simulink model "model_mavic_attitude_pid"  (R2020b)
settings: Solver=VariableStepAuto  StartTime=0.0  StopTime=10.0  RelTol=1e-3
libraries: pid_lib x1
settings Model: Creator=boringtao  LastModifiedBy=boringtao

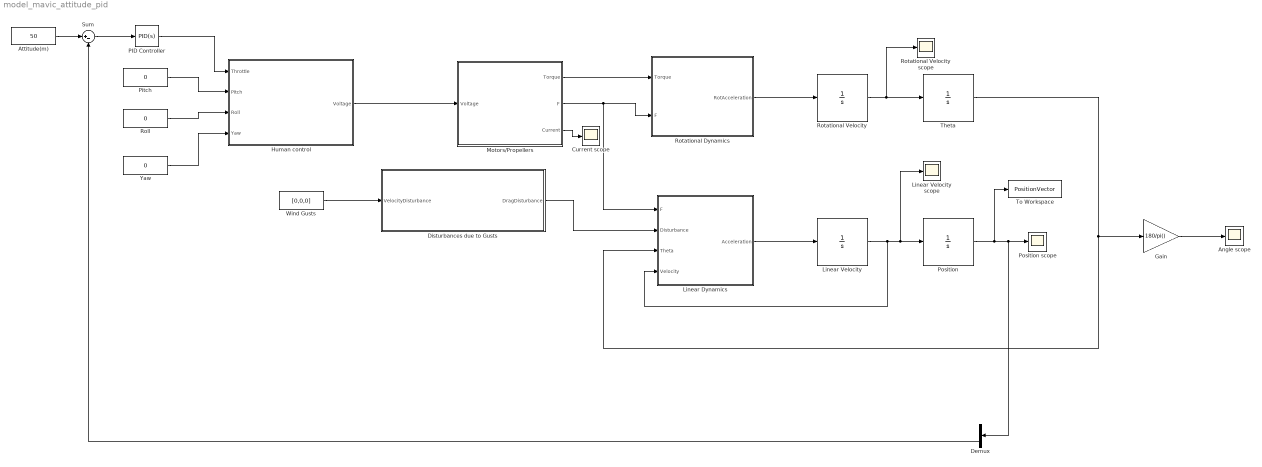
== system model_mavic_attitude_pid ==
  Angle scope : Scope
  Attitude(m) : Constant  Value=50
  Current scope : Scope
  Demux : Demux  Outputs=3
  Disturbances due to Gusts : MATLAB Function  TreatAsAtomicUnit=on
  Gain : Gain  Gain=180/pi()
  Human control : MATLAB Function  TreatAsAtomicUnit=on
  Linear Dynamics : MATLAB Function  TreatAsAtomicUnit=on
  Linear Velocity : Integrator
  Linear Velocity scope : Scope
  Motors/Propellers : MATLAB Function  TreatAsAtomicUnit=on
  PID Controller : pid_lib/PID Controller  Controller=PID  Form=Parallel  TimeDomain=Continuous-time  UseExternalTs=off  SampleTime=-1  IntegratorMethod=Forward Euler  FilterMethod=Forward Euler  ControllerParametersSource=internal  P=9.03216330858069  I=0.526929984868094  D=34.3994596994787  UseFilter=on  N=1142.8279760416  TunerSelectOption=Transfer Function Based (PID Tuner App)  InitialConditionSource=internal  InitialConditionForIntegrator=0  InitialConditionForFilter=0  DifferentiatorICPrevScaledInput=0  ExternalReset=none  TrackingMode=off  Kt=1  LimitOutput=on  SatLimitsSource=internal  UpperSaturationLimit=100  LowerSaturationLimit=0  LinearizeAsGain=on  AntiWindupMode=clamping  Kb=1  POutMin=[]  POutMax=[]  IOutMin=[]  IOutMax=[]  DOutMin=[]  DOutMax=[]  NOutMin=[]  NOutMax=[]  SumOutMin=[]  SumOutMax=[]  SaturationOutMin=[]  SaturationOutMax=[]  PParamMin=[]  PParamMax=[]  IParamMin=[]  IParamMax=[]  DParamMin=[]  DParamMax=[]  NParamMin=[]  NParamMax=[]  KbParamMin=[]  KbParamMax=[]  KtParamMin=[]  KtParamMax=[]  KbOutMin=[]  KbOutMax=[]  KtOutMin=[]  KtOutMax=[]  IntegratorOutMin=[]  IntegratorOutMax=[]  FilterOutMin=[]  FilterOutMax=[]  SumI1OutMin=[]  SumI1OutMax=[]  SumI2OutMin=[]  SumI2OutMax=[]  SumI3OutMin=[]  SumI3OutMax=[]  SumI4OutMin=[]  SumI4OutMax=[]  SumDOutMin=[]  SumDOutMax=[]  DifferentiatorOutMin=[]  DifferentiatorOutMax=[]  FilterDiffOutCoefMin=[]  FilterDiffOutCoefMax=[]  ReciprocalOutMin=[]  ReciprocalOutMax=[]  SumDenOutMin=[]  SumDenOutMax=[]  SumNumOutMin=[]  SumNumOutMax=[]  DivideOutMin=[]  DivideOutMax=[]  UdiffTsProdOutMin=[]  UdiffTsProdOutMax=[]  NTsProdOutMin=[]  NTsProdOutMax=[]  UintegralTsProdOutMin=[]  UintegralTsProdOutMax=[]  UngainTsProdOutMin=[]  UngainTsProdOutMax=[]  IntegratorContinuousStateAttributes=''  IntegratorStateMustResolveToSignalObject=off  IntegratorRTWStateStorageClass=Auto  FilterContinuousStateAttributes=''  FilterStateMustResolveToSignalObject=off  FilterRTWStateStorageClass=Auto  ParallelPVariant=InternalParameters  IdealPVariant=Disabled  IVariant=InternalParameters  DVariant=InternalParameters  IntegratorVariant=Continuous  SatVariant=Enabled  AWVariant=ContClampingParallel  PCopyVariant=Disabled  TRVariant=Disabled  FdbkBlocksVariant=Forward  IdealPFdbkVariant=Disabled  SatFdbkVariant=Disabled  DerivativeFilterVariant=ContFilter  NVariant=InternalParameters  NCopyVariant=Disabled  FilterICVariant=InternalICsFilter  IntegratorICVariant=InternalICs  ExternalResetVariant=Disabled  TRSumVariant=Passthrough  SumFdbkVariant=Disabled  SumVariant=Sum_PID  TsampFilterVariant=InternalTs  TsampNgainVariant=Passthrough  TsampIntegralVariant=Passthrough  ExternalSaturationOutDataTypeStr=Inherit: Same as second input
  Pitch : Constant  Value=0
  Position : Integrator
  Position scope : Scope
  Roll : Constant  Value=0
  Rotational Dynamics : MATLAB Function  TreatAsAtomicUnit=on
  Rotational Velocity : Integrator
  Rotational Velocity scope : Scope
  Sum : Sum  Inputs=|+-
  Theta : Integrator
  To Workspace : ToWorkspace  VariableName=PositionVector  SampleTime=-1
      settings: Save2DSignal=2-D array (concatenate along first dimension)
  Wind Gusts : Constant  Value=[0,0,0]
  Yaw : Constant  Value=0
  wires:
  Motors/Propellers/1(Torque) -> Rotational Dynamics/1(Torque)
  Motors/Propellers/2(F) -> Rotational Dynamics/2(F), Linear Dynamics/1(F)
  Rotational Dynamics/1(RotAcceleration) -> Rotational Velocity/1
  Rotational Velocity/1 -> Rotational Velocity scope/1, Theta/1
  Theta/1 -> Gain/1, Linear Dynamics/3(Theta)
  Linear Dynamics/1(Acceleration) -> Linear Velocity/1
  Linear Velocity/1 -> Linear Dynamics/4(Velocity), Linear Velocity scope/1, Position/1
  Disturbances due to Gusts/1(DragDisturbance) -> Linear Dynamics/2(Disturbance)
  Wind Gusts/1 -> Disturbances due to Gusts/1(VelocityDisturbance)
  Human control/1(Voltage) -> Motors/Propellers/1(Voltage)
  Position/1 -> To Workspace/1, Demux/1, Position scope/1
  Gain/1 -> Angle scope/1
  PID Controller/1 -> Human control/1(Throttle)
  Pitch/1 -> Human control/2(Pitch)
  Roll/1 -> Human control/3(Roll)
  Yaw/1 -> Human control/4(Yaw)
  Motors/Propellers/3(Current) -> Current scope/1
  Sum/1 -> PID Controller/1
  Attitude(m)/1 -> Sum/1
  Demux/3 -> Sum/2

== matlab function model_mavic_attitude_pid/Rotational Dynamics ==
  data: Torque input; RotAcceleration output; F input
function RotAcceleration = fcn(Torque, F)
Moment = [0 0 0];
RotAcceleration = [0 0 0];
I = [0.003 0.003 0.007];

Moment(1) = (F(3) + F(4))*0.237/2 - (F(1) + F(2))*0.237/2
Moment(2) = (F(3) + F(2))*0.237/2 - (F(1) + F(4))*0.237/2
Moment(3) = Torque(4) - Torque(1) + Torque(2) - Torque(4)

for i = 1:3
    RotAcceleration(i) = Moment(i)/I(i);
end

== matlab function model_mavic_attitude_pid/Motors//Propellers ==
  data: Voltage input; Torque output; F output; Current output
function [Torque, F, Current] = fcn(Voltage)
RPM = [0 0 0 0]
Torque = [0 0 0 0]
Current = [0 0 0 0]
F = [0 0 0 0]

for i=1:4
    RPM(i) = -2.6932*Voltage(i)^3 + 1400*Voltage(i);
    Ct = 2*10^ - 15*RPM(i)^3 - 4*10^ - 11*RPM(i)^2 + 3*10^ - 7*RPM(i) + 0.1013;
    F(i) = Ct*1.225*(RPM(i)/60)^2*0.2^4;
    Torque(i) = 4*10^ -14*RPM(i)^3 + 8*10^ -12*RPM(i)^2 + 3*10^ -6*RPM(i);
    Current(i) = 1400*Torque(i);
end

== matlab function model_mavic_attitude_pid/Linear Dynamics ==
  data: F input; Acceleration output; Disturbance input; Theta input; Velocity input
function Acceleration = fcn(F, Disturbance, Theta, Velocity)
m = 0.743;
g = 9.81;
A = [0.0197, 0.0197, 0.0512];
rho = 1.225;
Cd = 1;

Acceleration = [0 0 0];
Force = [0 0 0];
Fprop = [0 0 0];

Fprop(1) = sin(Theta(2))*cos(Theta(1))*(F(1)+F(2)+F(3)+F(4));
Fprop(2) = sin(Theta(1))*cos(Theta(2))*(F(1)+F(2)+F(3)+F(4));
Fprop(3) = cos(Theta(2))*cos(Theta(1))*(F(1)+F(2)+F(3)+F(4));

ThetaXY = -atan2(Fprop(1), Fprop(2));
XY2D = sqrt(Fprop(1)^2 + Fprop(2)^2);

if Fprop(3)>=0
    Fprop(1) = XY2D*sin(ThetaXY + Theta(3));
    Fprop(2) = XY2D*cos(ThetaXY + Theta(3));
else
    Fprop(1) = XY2D*sin(-ThetaXY + Theta(3));
    Fprop(2) = XY2D*cos(-ThetaXY + Theta(3));
end

if Velocity(1)<0
    Force(1)=Fprop(1)-Disturbance(1)+0.5*rho*Velocity(1)^2*A(1)*Cd;
else
    Force(1)=Fprop(1)-Disturbance(1)-0.5*rho*Velocity(1)^2*A(1)*Cd;
end

if Velocity(2)<0
    Force(2)=Fprop(2)-Disturbance(2)+0.5*rho*Velocity(2)^2*A(2)*Cd;
else
    Force(2)=Fprop(2)-Disturbance(2)-0.5*rho*Velocity(2)^2*A(2)*Cd;
end

if Velocity(3)<0
    Force(3)=Fprop(3)-Disturbance(3)+0.5*rho*Velocity(3)^2*A(3)*Cd-m*g;
else
    Force(3)=Fprop(3)-Disturbance(3)-0.5*rho*Velocity(3)^2*A(3)*Cd-m*g;
end

for i=1:3
    Acceleration(i)=Force(i)/m;
end

== matlab function model_mavic_attitude_pid/Disturbances due to Gusts ==
  data: VelocityDisturbance input; DragDisturbance output
function DragDisturbance = fcn(VelocityDisturbance)
A=[0.0197 0.0197 0.0197*2*1.3];
DragDisturbance = [0 0 0];
rho = 1.225;
Cd = 1;

for i=1:3
    if VelocityDisturbance(i)<0
        DragDisturbance(i) = 0.5*rho*VelocityDisturbance(i)^2*A(i)*Cd
    else
        DragDisturbance(i) = -0.5*rho*VelocityDisturbance(i)^2*A(i)*Cd
    end
end

== matlab function model_mavic_attitude_pid/Human control ==
  data: Throttle input; Voltage output; Pitch input; Roll input; Yaw input
function Voltage = fcn(Throttle, Pitch, Roll, Yaw)
Correct = 0;

if (Pitch/2+Roll/2+Yaw/2)>(100-Throttle)
    Correct = (Pitch/2+Roll/2+Yaw/2) - (100-Throttle);
end

if (Pitch/2+Roll/2+Yaw/2)<Throttle
    if Correct < ((Pitch/2+Roll/2+Yaw/2) - Throttle)
        Correct = (Pitch/2+Roll/2+Yaw/2) - Throttle;
    end
end

if Correct~=0
    Pitch = Pitch - Correct/3*2;
    Roll = Roll - Roll/3*2;
    Yaw = Yaw- Yaw/3*2;
end

Voltage = [(Throttle-Pitch/2-Roll/2-Yaw/2)*11.4/100
    (Throttle-Pitch/2+Roll/2+Yaw/2)*11.4/100
    (Throttle+Pitch/2+Roll/2-Yaw/2)*11.4/100
    (Throttle+Pitch/2-Roll/2+Yaw/2)*11.4/100];
